simulink library "dlbsBlockAdam"  (R2025b)
settings: Solver=VariableStepAuto  StartTime=0.0  StopTime=10.0  RelTol=1e-3
undefined symbols (not defined in the file or in its folder): DiscIntNeverNeededParam
libraries: dlbsBlockExtractGradientGF x1
settings Model: Creator=lt6037  LastModifiedBy=lt6037

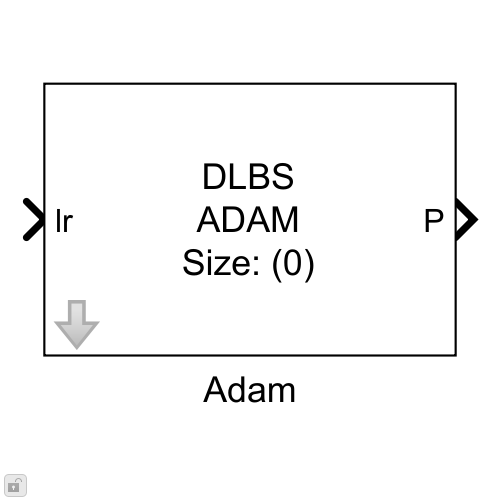
[thumbnail: Simulink's stored preview of the top-level diagram]
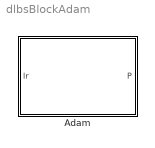
== system dlbsBlockAdam ==
  Adam : Subsystem  mask{init=randn(1,1), beta1=0.9, beta2=0.999, epsilon=1e-8}
      mask prompts: init "Initial Values"; beta1 "Beta 1"; beta2 "Beta 2"
      mask help:
      | Updates parameters using the Adam optimization algorithm.
      | Learnable parameters are owned by the optimizer. The output parameter tensor P is created and sized according to the init parameter.
      mask Help: web("dlbsHelpBlockAdam.html")
      mask Display:
      | try
      |     maskWs = Simulink.Mask.get(gcb).getWorkspace();
      |     sizeArray = size(maskWs.get("init"));
      | catch
      |     sizeArray = 0;
      | end
      | 
      | sizeString="(";
      | 
      | for k = 1:length(sizeArray)
      |     sizeString = sizeString+num2str(sizeArray(k));
      |     if k < length(sizeArray)
      |         sizeString = sizeString + ",";
      |     end
      | end
      | sizeString = sizeString + ")";
      | 
      | 
      | fprintf("DLBS\nADAM\nSize: %s",sizeString)

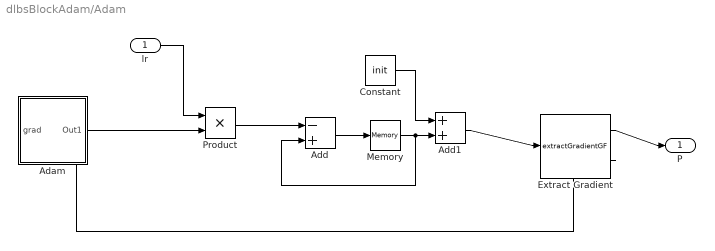
== system dlbsBlockAdam/Adam ==
  lr : Inport
  Adam : Subsystem
  Add : Sum  Inputs=-+
  Add1 : Sum
  Constant : Constant  Value=init  VectorParams1D=off
  Extract Gradient : dlbsBlockExtractGradientGF/extractGradientGF
  Memory : Memory  InitialCondition=zeros(size(init))  InheritSampleTime=on
  Product : Product
  P : Outport
  wires:
  Product/1 -> Add/1
  Add1/1 -> Extract Gradient/1
  Adam/1(Out1) -> Product/2
  Memory/1 -> Add1/2, Add/2
  Constant/1 -> Add1/1
  Add/1 -> Memory/1
  lr/1 -> Product/1
  Extract Gradient/2 -> Adam/1(grad)
  Extract Gradient/1 -> P/1

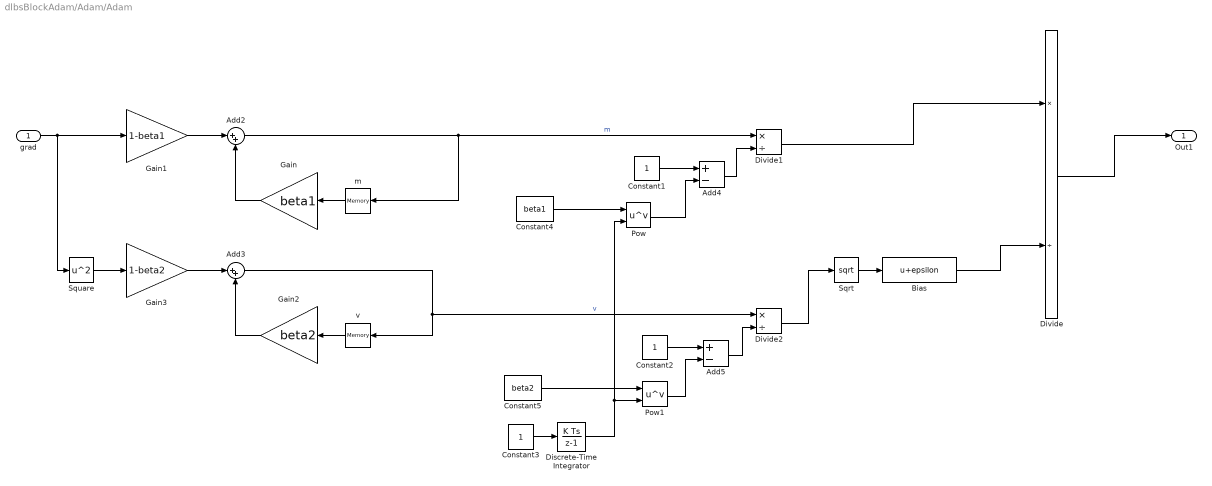
== system dlbsBlockAdam/Adam/Adam ==
  grad : Inport
  Add2 : Sum  Inputs=|++
  Add3 : Sum  Inputs=|++
  Add4 : Sum  Inputs=+-
  Add5 : Sum  Inputs=+-
  Bias : Bias  Bias=epsilon  SaturateOnIntegerOverflow=off
  Constant1 : Constant
  Constant2 : Constant
  Constant3 : Constant
  Constant4 : Constant  Value=beta1
  Constant5 : Constant  Value=beta2
  Discrete-Time Integrator : DiscreteIntegrator  InitialCondition=1  SampleTime=-1  ICPrevOutput=DiscIntNeverNeededParam  ICPrevScaledInput=DiscIntNeverNeededParam
  Divide : Product  Inputs=*/
  Divide1 : Product  Inputs=*/
  Divide2 : Product  Inputs=*/
  Gain : Gain  Gain=beta1
  Gain1 : Gain  Gain=1-beta1
  Gain2 : Gain  Gain=beta2
  Gain3 : Gain  Gain=1-beta2
  Pow : Math  Operator=pow  RndMeth=Zero
  Pow1 : Math  Operator=pow  RndMeth=Zero
  Sqrt : Sqrt
  Square : Math  Operator=square
  m : Memory  InitialCondition=zeros(size(init))  InheritSampleTime=on
  v : Memory  InitialCondition=zeros(size(init))  InheritSampleTime=on
  Out1 : Outport
  wires:
  Add5/1 -> Divide2/2
  m/1 -> Gain/1
  Divide/1 -> Out1/1
  Constant3/1 -> Discrete-Time Integrator/1
  Constant5/1 -> Pow1/1
  Add3/1 -> v/1, Divide2/1  "v"
  Constant1/1 -> Add4/1
  Constant2/1 -> Add5/1
  Constant4/1 -> Pow/1
  Gain2/1 -> Add3/2
  Gain1/1 -> Add2/1
  Pow/1 -> Add4/2
  Add4/1 -> Divide1/2
  Sqrt/1 -> Bias/1
  Pow1/1 -> Add5/2
  Discrete-Time Integrator/1 -> Pow/2, Pow1/2
  Add2/1 -> m/1, Divide1/1  "m"
  Square/1 -> Gain3/1
  Bias/1 -> Divide/2
  Gain3/1 -> Add3/1
  Gain/1 -> Add2/2
  grad/1 -> Square/1, Gain1/1
  v/1 -> Gain2/1
  Divide1/1 -> Divide/1
  Divide2/1 -> Sqrt/1
